simulink model "Decode_Encode_Analog"  (R2017a)
settings: Solver=VariableStepAuto  StartTime=0.0  StopTime=10  RelTol=1e-3
libraries: dsparch4 x3
settings Model: Creator=telep  LastModifiedBy=telep

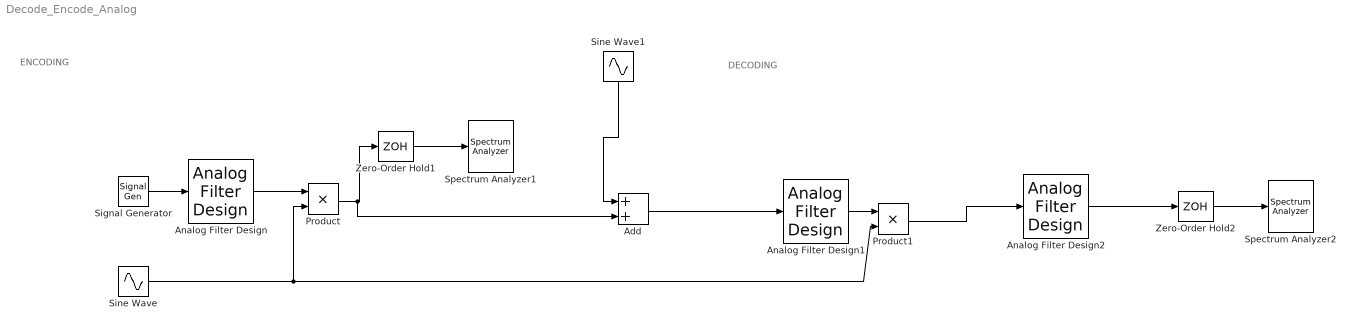
== system Decode_Encode_Analog ==
  note: DECODING
  note: ENCODING
  Add : Sum
  Analog Filter Design : dsparch4/Analog Filter Design  method=Butterworth  filttype=Lowpass  N=10  Wlo=2*3.14159*12800  Whi=80  Rp=2  Rs=40
  Analog Filter Design1 : dsparch4/Analog Filter Design  method=Butterworth  filttype=Lowpass  N=10  Wlo=2*3.14159*12800  Whi=80  Rp=2  Rs=40
  Analog Filter Design2 : dsparch4/Analog Filter Design  method=Butterworth  filttype=Lowpass  N=10  Wlo=2*3.14159*12800  Whi=80  Rp=2  Rs=40
  Product : Product
  Product1 : Product
  Signal Generator : SignalGenerator  WaveForm=square  Frequency=1/0.002
  Sine Wave : Sin  Amplitude=2  Frequency=2*3.14159*14000  SampleTime=0
  Sine Wave1 : Sin  Amplitude=2  Frequency=2*3.14159*750  SampleTime=0
  Spectrum Analyzer1 : SpectrumAnalyzer
  Spectrum Analyzer2 : SpectrumAnalyzer
  Zero-Order Hold1 : ZeroOrderHold  SampleTime=0.00001
  Zero-Order Hold2 : ZeroOrderHold  SampleTime=0.00001
  wires:
  Analog Filter Design/1 -> Product/1
  Sine Wave/1 -> Product1/2, Product/2
  Signal Generator/1 -> Analog Filter Design/1
  Product/1 -> Add/2, Zero-Order Hold1/1
  Zero-Order Hold1/1 -> Spectrum Analyzer1/1
  Analog Filter Design1/1 -> Product1/1
  Product1/1 -> Analog Filter Design2/1
  Zero-Order Hold2/1 -> Spectrum Analyzer2/1
  Analog Filter Design2/1 -> Zero-Order Hold2/1
  Add/1 -> Analog Filter Design1/1
  Sine Wave1/1 -> Add/1
